simulink model "Direct_MRAC_Simulink_Edition"  (R2018b)
settings: Solver=VariableStepAuto  StartTime=0.0  StopTime=30  RelTol=1e-3
settings Model: Creator=Bella  LastModifiedBy=Bella

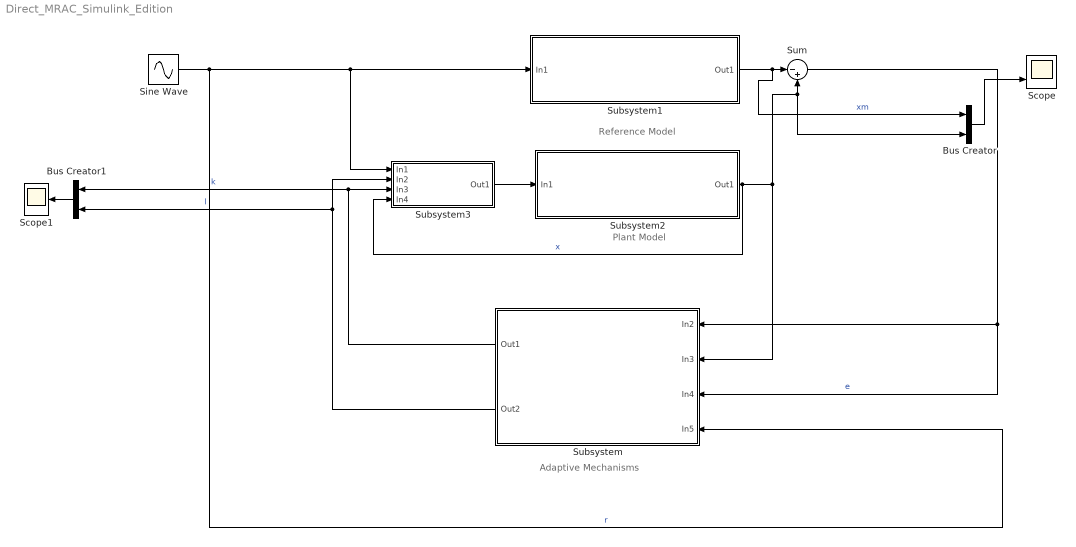
== system Direct_MRAC_Simulink_Edition ==
  note: Adaptive Mechanisms
  note: Plant Model
  note: Reference Model
  Bus Creator : BusCreator  Inputs=2
  Bus Creator1 : BusCreator  Inputs=2
  Scope : Scope  NumInputPorts=2
  Scope1 : Scope
  Sine Wave : Sin  Amplitude=2  Frequency=0.2  SampleTime=0
  Subsystem : Subsystem
  Subsystem1 : Subsystem  Description=Reference Model
  Subsystem2 : Subsystem
  Subsystem3 : Subsystem
  Sum : Sum  Inputs=|-+
  wires:
  Sine Wave/1 -> Subsystem1/1(In1), Subsystem3/1(In1), Subsystem/4(In5)  "r"
  Subsystem1/1(Out1) -> Bus Creator/1, Sum/1  "xm"
  Sum/1 -> Subsystem/3(In4), Subsystem/1(In2)  "e"
  Subsystem2/1(Out1) -> Subsystem3/4(In4), Bus Creator/2, Sum/2, Subsystem/2(In3)  "x"
  Subsystem3/1(Out1) -> Subsystem2/1(In1)
  Subsystem/1(Out1) -> Bus Creator1/1, Subsystem3/3(In3)  "k"
  Subsystem/2(Out2) -> Bus Creator1/2, Subsystem3/2(In2)  "l"
  Bus Creator/1 -> Scope/2
  Bus Creator1/1 -> Scope1/1

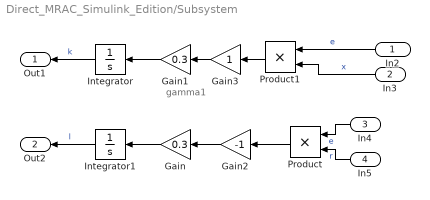
== system Direct_MRAC_Simulink_Edition/Subsystem ==
  note: gamma1
  In2 : Inport
  In3 : Inport  Port=2
  In4 : Inport  Port=3
  In5 : Inport  Port=4
  Gain : Gain  Gain=0.3
  Gain1 : Gain  Gain=0.3
  Gain2 : Gain  Gain=-1
  Gain3 : Gain
  Integrator : Integrator
  Integrator1 : Integrator
  Product : Product
  Product1 : Product
  Out1 : Outport
  Out2 : Outport  Port=2
  wires:
  Gain1/1 -> Integrator/1
  In2/1 -> Product1/1  "e"
  Gain/1 -> Integrator1/1
  In4/1 -> Product/1  "e"
  In3/1 -> Product1/2  "x"
  In5/1 -> Product/2  "r"
  Integrator/1 -> Out1/1  "k"
  Integrator1/1 -> Out2/1  "l"
  Gain2/1 -> Gain/1
  Product/1 -> Gain2/1
  Gain3/1 -> Gain1/1
  Product1/1 -> Gain3/1

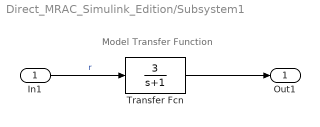
== system Direct_MRAC_Simulink_Edition/Subsystem1 ==
  note: Model Transfer Function
  In1 : Inport
  Transfer Fcn : TransferFcn  Numerator=[3]  Denominator=[1 1]
  Out1 : Outport
  wires:
  In1/1 -> Transfer Fcn/1  "r"
  Transfer Fcn/1 -> Out1/1

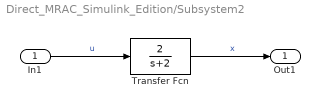
== system Direct_MRAC_Simulink_Edition/Subsystem2 ==
  In1 : Inport
  Transfer Fcn : TransferFcn  Numerator=[2]  Denominator=[1 2]
  Out1 : Outport
  wires:
  In1/1 -> Transfer Fcn/1  "u"
  Transfer Fcn/1 -> Out1/1  "x"

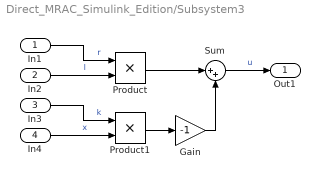
== system Direct_MRAC_Simulink_Edition/Subsystem3 ==
  In1 : Inport
  In2 : Inport  Port=2
  In3 : Inport  Port=3
  In4 : Inport  Port=4
  Gain : Gain  Gain=-1
  Product : Product
  Product1 : Product
  Sum : Sum  Inputs=|++
  Out1 : Outport
  wires:
  In1/1 -> Product/1  "r"
  In2/1 -> Product/2  "l"
  In3/1 -> Product1/1  "k"
  In4/1 -> Product1/2  "x"
  Product/1 -> Sum/1
  Sum/1 -> Out1/1  "u"
  Product1/1 -> Gain/1
  Gain/1 -> Sum/2
